simulink model "version2"  (R2021a)
settings: Solver=VariableStepAuto  StartTime=0.0  StopTime=10.0  RelTol=1e-3
settings Model: Creator=danesh  LastModifiedBy=danesh

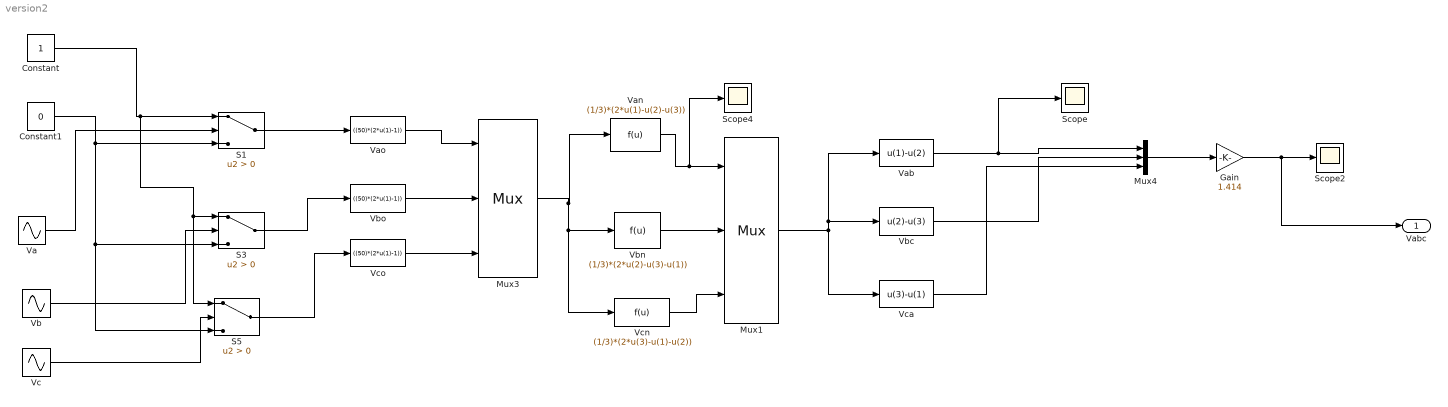
== system version2 ==
  Constant : Constant
  Constant1 : Constant  Value=0
  Gain : Gain  Gain=1.414
  Mux1 : Mux  Inputs=3
  Mux3 : Mux  Inputs=3
  Mux4 : Mux  Inputs=3
  S1 : Switch  Criteria=u2 > Threshold
  S3 : Switch  Criteria=u2 > Threshold
  S5 : Switch  Criteria=u2 > Threshold
  Scope : Scope
  Scope2 : Scope
  Scope4 : Scope
  Va : Sin  Frequency=2*pi*50  SampleTime=0
  Vab : Fcn  Expr=u(1)-u(2)
  Van : Fcn  Expr=(1/3)*(2*u(1)-u(2)-u(3))
  Vao : Fcn  Expr=((50)*(2*u(1)-1))
  Vb : Sin  Frequency=2*pi*50  Phase=-2.0904  SampleTime=0
  Vbc : Fcn  Expr=u(2)-u(3)
  Vbn : Fcn  Expr=(1/3)*(2*u(2)-u(3)-u(1))
  Vbo : Fcn  Expr=((50)*(2*u(1)-1))
  Vc : Sin  Frequency=2*pi*50  Phase=-4.188  SampleTime=0
  Vca : Fcn  Expr=u(3)-u(1)
  Vcn : Fcn  Expr=(1/3)*(2*u(3)-u(1)-u(2))
  Vco : Fcn  Expr=((50)*(2*u(1)-1))
  Vabc : Outport  VectorParamsAs1DForOutWhenUnconnected=off
  wires:
  Vcn/1 -> Mux1/3
  Constant1/1 -> S1/3, S3/3, S5/3
  Mux4/1 -> Gain/1
  S1/1 -> Vao/1
  Vbc/1 -> Mux4/2
  Mux1/1 -> Vbc/1, Vab/1, Vca/1
  Vab/1 -> Scope/1, Mux4/1
  Mux3/1 -> Van/1, Vcn/1, Vbn/1
  Vao/1 -> Mux3/1
  Vc/1 -> S5/2
  Van/1 -> Scope4/1, Mux1/1
  Constant/1 -> S3/1, S5/1, S1/1
  S3/1 -> Vbo/1
  Vbn/1 -> Mux1/2
  Vca/1 -> Mux4/3
  Vco/1 -> Mux3/3
  Gain/1 -> Vabc/1, Scope2/1
  Vb/1 -> S3/2
  S5/1 -> Vco/1
  Vbo/1 -> Mux3/2
  Va/1 -> S1/2
